simulink model "receiver_BAK"  (R2021b)
settings: Solver=FixedStepAuto  StartTime=0  StopTime=1800  FixedStep=0.025  RelTol=1e-3
libraries: slpidlib x1, SignalEditorBlockLib x1, dspnetwork x1, slrealtimeiplib x1, slrealtimeutilitieslib x1
settings Model: Creator=kytol  LastModifiedBy=kytol
settings DataIOCC: SaveFormat=StructureWithTime
settings OptimizationCC: BlockReduction=off  BufferReuse=off
settings DebuggingCC: AlgebraicLoopMsg=none  UnconnectedInputMsg=none  UnconnectedOutputMsg=none  UnconnectedLineMsg=none

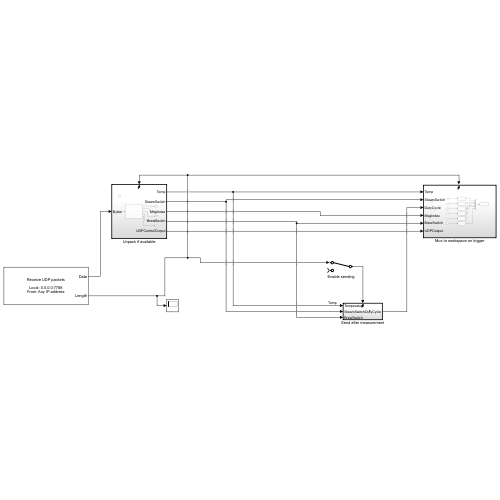
[thumbnail: Simulink's stored preview of the top-level diagram]
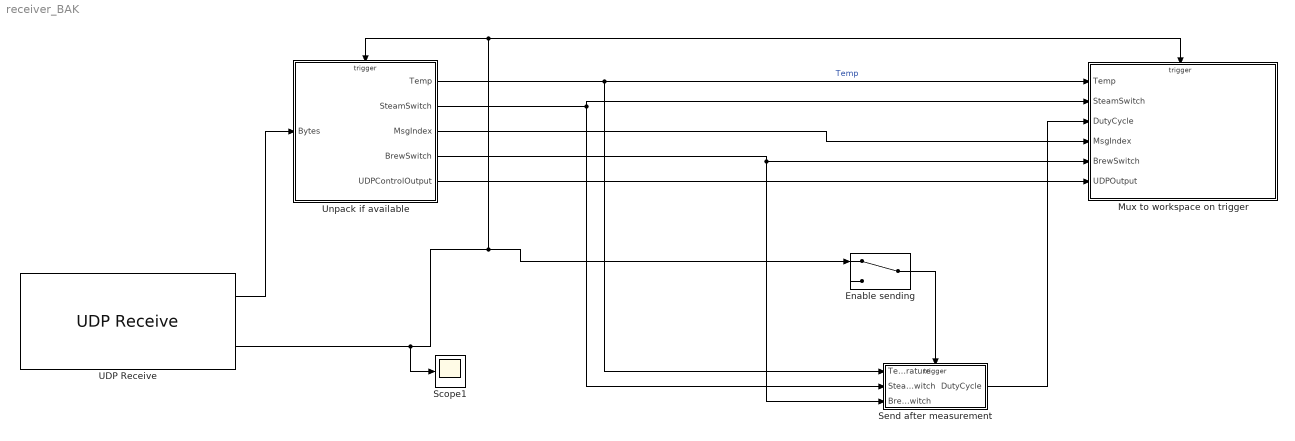
== system receiver_BAK ==
  Enable sending : ManualSwitch
  Mux to workspace on trigger : Subsystem
  Scope1 : Scope
  Send after measurement : Subsystem
  UDP Receive : slrealtimeiplib/UDP Receive  useHostTargetConn=off  ipAddress=0.0.0.0  localPort=7788  rcvWidth=14  rcvFmAny=on  fmAddress='10.10.10.10'  sampleTime=-1
      settings: SourceProductBaseCode=XP
  Unpack if available : Subsystem
  wires:
  UDP Receive/2 -> Scope1/1, Enable sending/1, Unpack if available/Trigger, Mux to workspace on trigger/Trigger
  UDP Receive/1 -> Unpack if available/1(Bytes)
  Unpack if available/1(Temp) -> Mux to workspace on trigger/1(Temp), Send after measurement/1(Temperature)  "Temp"
  Unpack if available/2(SteamSwitch) -> Mux to workspace on trigger/2(SteamSwitch), Send after measurement/2(SteamSwitch)
  Enable sending/1 -> Send after measurement/Trigger
  Send after measurement/1(DutyCycle) -> Mux to workspace on trigger/3(DutyCycle)
  Unpack if available/3(MsgIndex) -> Mux to workspace on trigger/4(MsgIndex)
  Unpack if available/4(BrewSwitch) -> Mux to workspace on trigger/5(BrewSwitch), Send after measurement/3(BrewSwitch)
  Unpack if available/5(UDPControlOutput) -> Mux to workspace on trigger/6(UDPOutput)

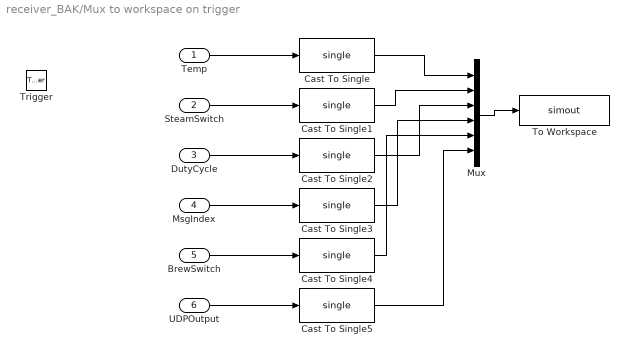
== system receiver_BAK/Mux to workspace on trigger ==
  Temp : Inport
  SteamSwitch : Inport  Port=2
  DutyCycle : Inport  Port=3
  MsgIndex : Inport  Port=4
  BrewSwitch : Inport  Port=5
  UDPOutput : Inport  Port=6
  Trigger : TriggerPort  VariantControl=(inherit)  PortDimensions=1
  Cast To Single{,1..5} (6 alike) : DataTypeConversion  OutDataTypeStr=single
  Mux : Mux  Inputs=6
  To Workspace : ToWorkspace  VariableName=simout  SaveFormat=Timeseries  SampleTime=-1
  wires:
  Temp/1 -> Cast To Single/1
  Mux/1 -> To Workspace/1
  Cast To Single2/1 -> Mux/3
  Cast To Single1/1 -> Mux/2
  Cast To Single/1 -> Mux/1
  SteamSwitch/1 -> Cast To Single1/1
  DutyCycle/1 -> Cast To Single2/1
  MsgIndex/1 -> Cast To Single3/1
  Cast To Single3/1 -> Mux/4
  BrewSwitch/1 -> Cast To Single4/1
  Cast To Single4/1 -> Mux/5
  UDPOutput/1 -> Cast To Single5/1
  Cast To Single5/1 -> Mux/6

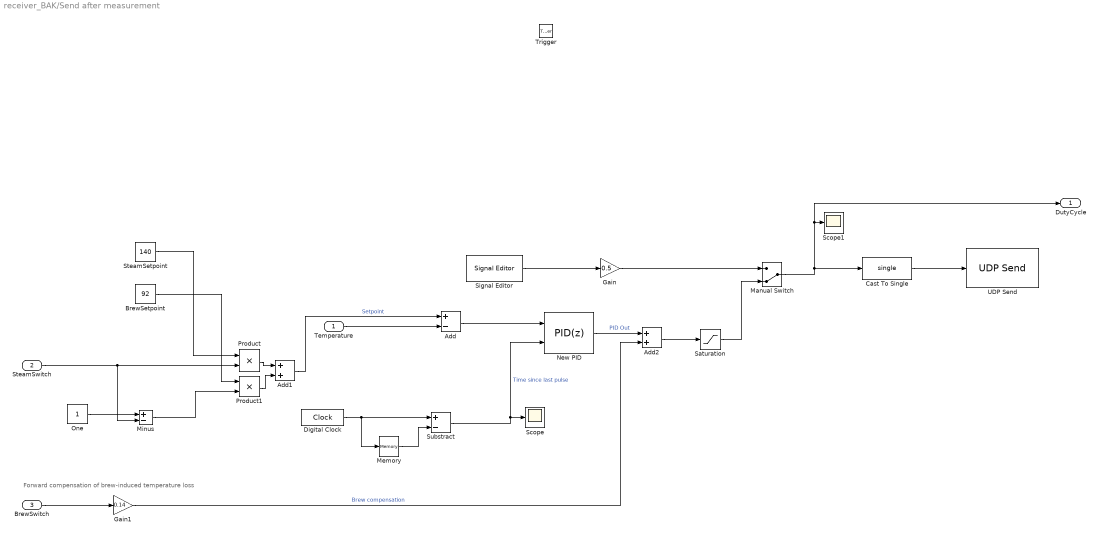
== system receiver_BAK/Send after measurement ==
  note: Forward compensation of brew-induced temperature loss
  Temperature : Inport
  SteamSwitch : Inport  Port=2
  BrewSwitch : Inport  Port=3
  Trigger : TriggerPort  VariantControl=(inherit)  PortDimensions=1
  Add : Sum  Inputs=+-
  Add1 : Sum
  Add2 : Sum
  BrewSetpoint : Constant  Value=92
  Cast To Single : DataTypeConversion  OutDataTypeStr=single
  Digital Clock : DigitalClock  SampleTime=-1
  Gain : Gain  Gain=0.5
  Gain1 : Gain  Gain=0.14
  Manual Switch : ManualSwitch  CurrentSetting=0
  Memory : Memory  InheritSampleTime=on  LinearizeAsDelay=on
  Minus : Sum  Inputs=+-
  New PID : slpidlib/PID Controller  Controller=PID  Form=Parallel  TimeDomain=Discrete-time  UseExternalTs=on  SampleTime=0.5  IntegratorMethod=Forward Euler  FilterMethod=Forward Euler  ControllerParametersSource=internal  P=0.046  I=0.0018  D=-0.0030  UseFilter=on  N=3.16854404448094  TunerSelectOption=Transfer Function Based (PID Tuner App)  ZeroCross=off  InitialConditionSource=internal  InitialConditionForIntegrator=0  InitialConditionForFilter=0  DifferentiatorICPrevScaledInput=0  ExternalReset=none  TrackingMode=off  Kt=1  LimitOutput=on  SatLimitsSource=internal  UpperSaturationLimit=1  LowerSaturationLimit=0  LinearizeAsGain=off  AntiWindupMode=clamping  Kb=1  POutMin=[]  POutMax=[]  IOutMin=[]  IOutMax=[]  DOutMin=[]  DOutMax=[]  NOutMin=[]  NOutMax=[]  SumOutMin=[]  SumOutMax=[]  SaturationOutMin=[]  SaturationOutMax=[]  PParamMin=[]  PParamMax=[]  IParamMin=[]  IParamMax=[]  DParamMin=[]  DParamMax=[]  NParamMin=[]  NParamMax=[]  KbParamMin=[]  KbParamMax=[]  KtParamMin=[]  KtParamMax=[]  KbOutMin=[]  KbOutMax=[]  KtOutMin=[]  KtOutMax=[]  IntegratorOutMin=[]  IntegratorOutMax=[]  FilterOutMin=[]  FilterOutMax=[]  SumI1OutMin=[]  SumI1OutMax=[]  SumI2OutMin=[]  SumI2OutMax=[]  SumI3OutMin=[]  SumI3OutMax=[]  SumI4OutMin=[]  SumI4OutMax=[]  SumDOutMin=[]  SumDOutMax=[]  DifferentiatorOutMin=[]  DifferentiatorOutMax=[]  FilterDiffOutCoefMin=[]  FilterDiffOutCoefMax=[]  ReciprocalOutMin=[]  ReciprocalOutMax=[]  SumDenOutMin=[]  SumDenOutMax=[]  SumNumOutMin=[]  SumNumOutMax=[]  DivideOutMin=[]  DivideOutMax=[]  UdiffTsProdOutMin=[]  UdiffTsProdOutMax=[]  NTsProdOutMin=[]  NTsProdOutMax=[]  UintegralTsProdOutMin=[]  UintegralTsProdOutMax=[]  UngainTsProdOutMin=[]  UngainTsProdOutMax=[]  IntegratorContinuousStateAttributes=''  IntegratorStateMustResolveToSignalObject=off  IntegratorRTWStateStorageClass=Auto  FilterContinuousStateAttributes=''  FilterStateMustResolveToSignalObject=off  FilterRTWStateStorageClass=Auto  ParallelPVariant=InternalParameters  IdealPVariant=Disabled  IVariant=InternalParameters  DVariant=InternalParameters  IntegratorVariant=Discrete  SatVariant=Enabled  AWVariant=DiscClampingParallel  PCopyVariant=Disabled  TRVariant=Disabled  FdbkBlocksVariant=Forward  IdealPFdbkVariant=Disabled  SatFdbkVariant=Disabled  DerivativeFilterVariant=ForwardEulerFilter  NVariant=InternalParameters  NCopyVariant=Disabled  FilterICVariant=InternalICsFilter  IntegratorICVariant=InternalICs  ExternalResetVariant=Disabled  TRSumVariant=Passthrough  SumFdbkVariant=Disabled  SumVariant=Sum_PID  TsampFilterVariant=ExternalTs  TsampNgainVariant=ExternalTs  TsampIntegralVariant=ExternalTs  ExternalSaturationOutDataTypeStr=Inherit: Same as second input
  One : Constant  OutDataTypeStr=Inherit: Inherit via back propagation
  Product : Product
  Product1 : Product
  Saturation : Saturate  UpperLimit=1  LowerLimit=0
  Scope : Scope
  Scope1 : Scope
  Signal Editor : SignalEditorBlockLib/Signal Editor  FileName=testsignals.mat  ActiveScenario=Testsignal  ActiveSignal=SquareSawStep  IsBus=off  OutputBusObjectStr=Bus: BusObject  SampleTime=-1  ZeroCross=off  OutputAfterFinalValue=Setting to zero  Unit=inherit  PreserveSignalName=on
  SteamSetpoint : Constant  Value=140
  Substract : Sum  Inputs=+-
  UDP Send : dspnetwork/UDP Send  remoteURL='192.168.1.107'  remotePort=7788  localURL='0.0.0.0'  localPortSource=Automatically determine  localPort=-1  sendBufferSize=64  sampletime=-1  blockPlatform=HOST  separateLengthPort=0
  DutyCycle : Outport
  wires:
  Cast To Single/1 -> UDP Send/1
  Manual Switch/1 -> DutyCycle/1, Scope1/1, Cast To Single/1
  Signal Editor/1 -> Gain/1
  Gain/1 -> Manual Switch/1
  Temperature/1 -> Add/2
  Add/1 -> New PID/1
  Digital Clock/1 -> Substract/1, Memory/1
  Memory/1 -> Substract/2
  Substract/1 -> New PID/2, Scope/1  "Time since last pulse"
  SteamSetpoint/1 -> Product/1
  BrewSetpoint/1 -> Product1/1
  Product/1 -> Add1/1
  Product1/1 -> Add1/2
  Add1/1 -> Add/1  "Setpoint"
  SteamSwitch/1 -> Minus/2, Product/2
  One/1 -> Minus/1
  Minus/1 -> Product1/2
  BrewSwitch/1 -> Gain1/1
  Gain1/1 -> Add2/2  "Brew compensation"
  New PID/1 -> Add2/1  "PID Out"
  Add2/1 -> Saturation/1
  Saturation/1 -> Manual Switch/2

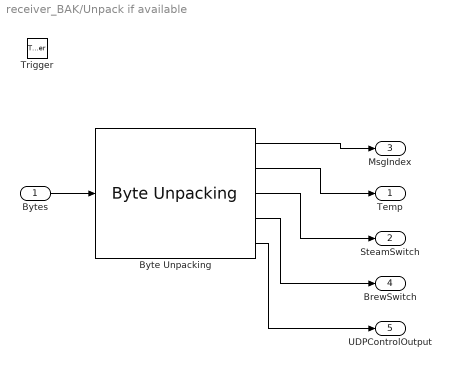
== system receiver_BAK/Unpack if available ==
  Bytes : Inport
  Trigger : TriggerPort  VariantControl=(inherit)  PortDimensions=1
  Byte Unpacking : slrealtimeutilitieslib/Byte Unpacking  MaskUnpackedDataTypes={'int32','single', 'int8', 'int8','single'}  MaskUnpackedDataSizes={[1],[1],[1],[1],[1]}  MaskAlignment=1
      settings: SourceProductBaseCode=XP
  Temp : Outport
  SteamSwitch : Outport  Port=2
  MsgIndex : Outport  Port=3
  BrewSwitch : Outport  Port=4
  UDPControlOutput : Outport  Port=5
  wires:
  Bytes/1 -> Byte Unpacking/1
  Byte Unpacking/3 -> SteamSwitch/1
  Byte Unpacking/2 -> Temp/1
  Byte Unpacking/1 -> MsgIndex/1
  Byte Unpacking/4 -> BrewSwitch/1
  Byte Unpacking/5 -> UDPControlOutput/1
